simulink model "AIE_HLS"  (R2023a)
settings: Solver=FixedStepDiscrete  StartTime=0.0  StopTime=100*2e-9  RelTol=1e-3
undefined symbols (not defined in the file): i, L, nsvg1369, xcvc1502
libraries: dspsrcs4 x3, aieBasic x3, hlsBasic x2, vmcUtilities x1
settings Model: Creator=shirazi  LastModifiedBy=robg
settings SolverCC: AlgebraicLoopSolver=TrustRegion
settings DebuggingCC: UnconnectedInputMsg=warning  UnconnectedOutputMsg=warning  UnconnectedLineMsg=warning
settings ModelReferenceCC: EnableRefExpFcnMdlSchedulingChecks=on
settings SFSimCC: CustomCodeUndefinedFunction=UseInterfaceOnly
settings RTWCC: DLArmComputeVersion=19.05

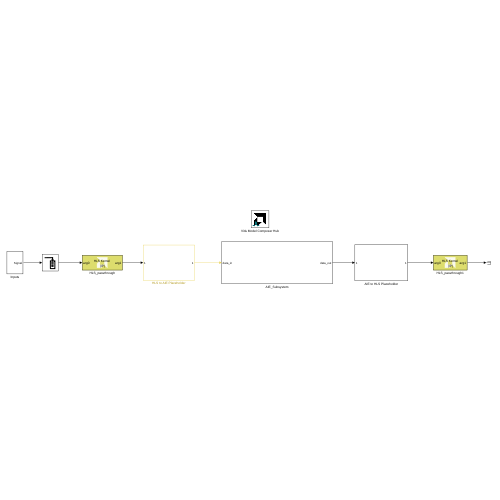
[thumbnail: Simulink's stored preview of the top-level diagram]
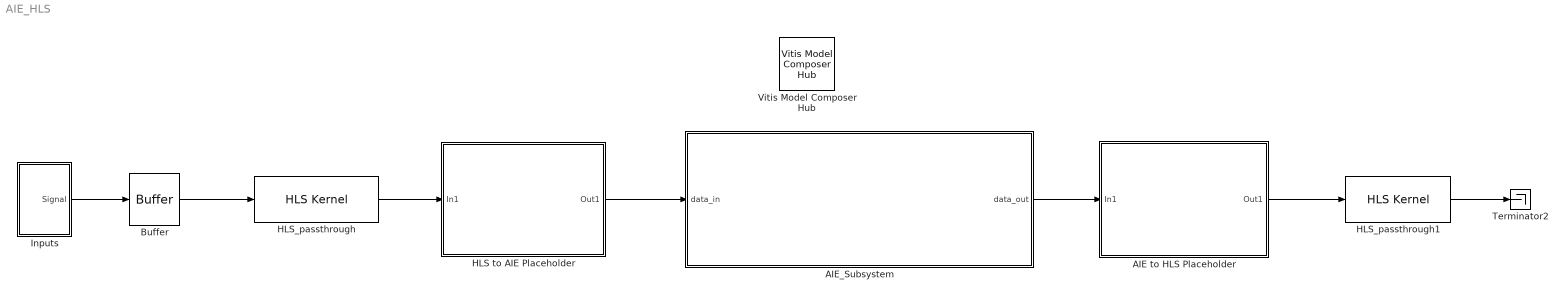
== system AIE_HLS ==
  AIE to HLS Placeholder : Subsystem
  AIE_Subsystem : Subsystem
  Buffer : Buffer  N=8  OutputFrames=off
  HLS to AIE Placeholder : Subsystem
  HLS_passthrough : hlsBasic/HLS Kernel  PortNames={'return'; 'arg0'; 'arg1'}  PortSerializedTypes={'{Bv}'; '{R{Thls::stream{2{t{Bu64t}}{t{}0}}}}'; '{R{Thls::stream{2{t{Bu64t}}{t{}0}}}}'}  FunctionTemplateSpecKind=none  FunctionTemplateParamNames={}  FunctionTemplateParamKinds={}  FunctionTemplateParamTypes={}  FunctionTemplateParamValues={}  PortSynchronicities={'auto'; 'auto'}  PortSignalSizes={0.000000000000000000e+00; 8.000000000000000000e+00}  PortParameterValues={}  FunctionTemplateParams={}  FunctionTemplateParamsEnables={}  FunctionTemplateParamsVisible=off  FunctionDeclTypeOptions=C[1 1]@t7@<empty>  PortAttributesTable={ 'Input', 'arg0', 'hls::stream< uint64_t, 0 > &', '', ''; 'Output', 'arg1', 'hls::stream< uint64_t, 0 > &', '', '8' }  PortAttributesEnablement={'off', 'off', 'off', 'off', 'off';'off', 'off', 'off', 'off', 'on'}  PortParametersTable={}  SampleTime=-1  PortDirectionTable={ 'arg0', 'hls::stream< uint64_t, 0 > &', 'Input', 'Port'; 'arg1', 'hls::stream< uint64_t, 0 > &', 'Output', 'Port' }  PortDirectionTabVisible=on  ArgDirections={1.000000000000000000e+00; 2.000000000000000000e+00}  ArgInterfaceTypes={1.000000000000000000e+00; 1.000000000000000000e+00}  FunctionIndex=1  FormalArgDecls={'hls::stream< uint64_t, 0 > & arg0', 'hls::stream< uint64_t, 0 > & arg1'}  SimLibPath=''  FunctionTabVisible=on  FunctionDescription=void HLS_passthrough(hls::stream< uint64_t, 0 > & arg0, hls::stream< uint64_t, 0 > & arg1)  blockJsonConstraints=[]  deprecateConstraints=0  KernelHeaderFile=HLS_passthrough.h  KernelFunction=HLS_passthrough  KernelFunctionSelect=<empty>  KernelSourceFile=HLS_passthrough.cpp  KernelSearchPaths={}  PreProcOptions={}
  HLS_passthrough1 : hlsBasic/HLS Kernel  PortNames={'return'; 'arg0'; 'arg1'}  PortSerializedTypes={'{Bv}'; '{R{Thls::stream{2{t{Bu64t}}{t{}0}}}}'; '{R{Thls::stream{2{t{Bu64t}}{t{}0}}}}'}  FunctionTemplateSpecKind=none  FunctionTemplateParamNames={}  FunctionTemplateParamKinds={}  FunctionTemplateParamTypes={}  FunctionTemplateParamValues={}  PortSynchronicities={'auto'; 'auto'}  PortSignalSizes={0.000000000000000000e+00; 8.000000000000000000e+00}  PortParameterValues={}  FunctionTemplateParams={}  FunctionTemplateParamsEnables={}  FunctionTemplateParamsVisible=off  FunctionDeclTypeOptions=C[1 1]@t7@<empty>  PortAttributesTable={ 'Input', 'arg0', 'hls::stream< uint64_t, 0 > &', '', ''; 'Output', 'arg1', 'hls::stream< uint64_t, 0 > &', '', '8' }  PortAttributesEnablement={'off', 'off', 'off', 'off', 'off';'off', 'off', 'off', 'off', 'on'}  PortParametersTable={}  SampleTime=-1  PortDirectionTable={ 'arg0', 'hls::stream< uint64_t, 0 > &', 'Input', 'Port'; 'arg1', 'hls::stream< uint64_t, 0 > &', 'Output', 'Port' }  PortDirectionTabVisible=on  ArgDirections={1.000000000000000000e+00; 2.000000000000000000e+00}  ArgInterfaceTypes={1.000000000000000000e+00; 1.000000000000000000e+00}  FunctionIndex=1  FormalArgDecls={'hls::stream< uint64_t, 0 > & arg0', 'hls::stream< uint64_t, 0 > & arg1'}  SimLibPath=''  FunctionTabVisible=on  FunctionDescription=void HLS_passthrough(hls::stream< uint64_t, 0 > & arg0, hls::stream< uint64_t, 0 > & arg1)  blockJsonConstraints=[]  deprecateConstraints=0  KernelHeaderFile=HLS_passthrough.h  KernelFunction=HLS_passthrough  KernelFunctionSelect=<empty>  KernelSourceFile=HLS_passthrough.cpp  KernelSearchPaths={}  PreProcOptions={}
  Inputs : Subsystem
  Terminator2 : Terminator
  Vitis Model Composer Hub : vmcUtilities/Vitis Model Composer Hub  Tag=genX  CodeGeneration=off  StartColumn=1  NumberOfColumns=1  TargetDirectory=./code  exportDesign=off  analyzeDesign=off  validateDesignOnHw=off  ExportType=AI Engines  IpVendor=xilinx.com  IpLibrary=hls  IpVersion=1.0  IpHWLanguage=Verilog  AieCompilerOptions={}  AieSimulatorOptions={}  CreateTestbench=off  TestbenchStackSize=10  RunRtlSim=off  RunCSim=off  RunAieSim=off  AieSimTimeout=50000  RunAieSimProfiling=off  LaunchVitisAnalyzer=off  PlotOutput=off  RunX86Sim=off  X86SimTimeout=10  GenHwImage=off  GenLibadfXo=off  GenHwValidationCode=off  PlatformType=Not Specified  HwSystemType=Baremetal  HwValidationTarget=hw  ProjDevice=xcvc1502-nsvg1369-1LHP-i-L  ProjDevicePart=xcvc1502-nsvg1369-1LHP-i-L  AIEType=AIE  SamplePeriod=-1  ClockFrequency=200  DataPathParallelism=1  xilinxfamily=versalaicore  part=xcvc1502  speed=-1LHP-i-L  package=nsvg1369  directory=./code  testbench=off  incr_netlist=off  synthesis_tool=Vivado  clock_wrapper=Clock Enables  dbl_ovrd=According to Block Masks  dcm_input_clock_period=10  sysclk_period=10  simulink_period=1  eval_field=0  LogFileName=''  NThreads=4
  wires:
  HLS to AIE Placeholder/1(Out1) -> AIE_Subsystem/1(data_in)
  AIE_Subsystem/1(data_out) -> AIE to HLS Placeholder/1(In1)
  Inputs/1(Signal) -> Buffer/1
  HLS_passthrough1/1 -> Terminator2/1
  AIE to HLS Placeholder/1(Out1) -> HLS_passthrough1/1
  HLS_passthrough/1 -> HLS to AIE Placeholder/1(In1)
  Buffer/1 -> HLS_passthrough/1

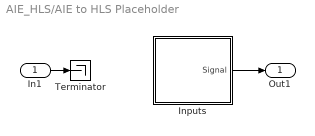
== system AIE_HLS/AIE to HLS Placeholder ==
  In1 : Inport
  Inputs : Subsystem
  Terminator : Terminator
  Out1 : Outport
  wires:
  Inputs/1(Signal) -> Out1/1
  In1/1 -> Terminator/1

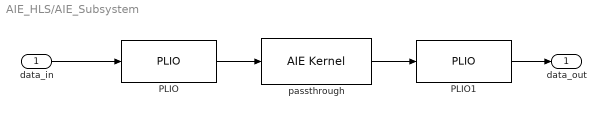
== system AIE_HLS/AIE_Subsystem ==
  data_in : Inport
  PLIO : aieBasic/PLIO  PlioWidth=64  PlioFreqSpec=on  PlioFreq=500  ColLocation=0  channel=0  blockJsonConstraints=[]  deprecateConstraints=0
  PLIO1 : aieBasic/PLIO  PlioWidth=64  PlioFreqSpec=on  PlioFreq=500  ColLocation=0  channel=0  blockJsonConstraints=[]  deprecateConstraints=0
  passthrough : aieBasic/AIE Kernel  KernelAllAttrs=|  PortNames={'in'; 'out'}  PortSerializedTypes={'{R{Tadf::input_buffer{1{t{Scint16}}}}}'; '{R{Tadf::output_buffer{1{t{Scint16}}}}}'}  PortWindowSizes={1.600000000000000000e+01, 1.600000000000000000e+01}  PortWindowMargins={0.000000000000000000e+00, 0.000000000000000000e+00}  PortSynchronicities={'sync', 'sync'}  PortSignalSizes={0.000000000000000000e+00; 0.000000000000000000e+00}  FunctionTemplateSpecKind=implicit  FunctionTemplateParamNames={'FRAME_LENGTH'}  FunctionTemplateParamKinds={'nontype'}  FunctionTemplateParamTypes={'int'}  FunctionTemplateParamValues={'16'}  FunctionIndex=1  FunctionTabVisible=on  FunctionTemplateParamsVisible=on  FunctionDeclTypeOptions=|  FunctionDecl=|  FunctionTemplateParams={ 'FRAME_LENGTH', 'int', '16' }  FunctionTemplateParamsEnables={'off', 'off', 'on'}  PortAttrs={ 'input', 'in', 'adf::input_buffer< cint16 > &', '16', '0', 'sync', ''; 'output', 'out', 'adf::output_buffer< cint16 > &', '16', '', 'sync', '' }  PortAttrsEnables={'off', 'off', 'off', 'on', 'off', 'off', 'off';'off', 'off', 'off', 'on', 'off', 'off', 'off'}  SampleTime=-1  KernelHeaderFile=passthrough.h  KernelFunction=passthrough  KernelSourceFile=passthrough.cc  KernelSearchPaths={}  PreProcOptions={}  blockJsonConstraints=[]
      KernelAllAttrs=|
      | s[12;12;9;9;19;14;21;23;21;23;24;21;15;17;12;24;26;26;26;27;28;9;21;23;23;23;24;25;14;19;19;29]@FunctionNameDeclFileNamePortNamesPortTypesPortSerializedTypesPortDirectionsPortWindowSizeEnablesPortWindowMarginEnablesPortBufferSizeEnablesPortBufferMarginEnablesPortSynchronicityEnablesPortSignalSizeEnablesPortBufferSizesPortBufferMarginsFunctionDeclFunctionTemplateSpecKindFunctionTemplateParamNamesFunctionTemplateParamKindsFunctionTemplateParamTypesFunctionTemplateParamValuesFunctionTemplateParamEnablesClassDeclClassTemplateSpecKindClassTemplateParamNamesClassTemplateParamKindsClassTemplateParamTypesClassTemplateParamValuesClassTemplateParamEnablesClassCtorDeclsClassCtorParamNamesClassCtorParamTypesClassCtorParamSerializedTypes[1 1]@C[32 1]@t11@passthrought19@../../passthrough.hC[2 1]@t2@int3@outC[2 1]@t29@adf::input_buffer< cint16 > &t30@adf::output_buffer< cint16 > &C[2 1]@t38@{R{Tadf::input_buffer{1{t{Scint16}}}}}t39@{R{Tadf::output_buffer{1{t{Scint16}}}}}C[2 1]@t5@inputt6@outputC[2 1]@l1@l1@C[2 1]@l1@l0@C[2 1]@l1@l1@C[2 1]@l0@l0@C[2 1]@l1@l1@C[2 1]@l0@l0@C[2 1]@nnC[2 1]@nnt117@template < int FRAME_LENGTH > 
      | void passthrough(adf::input_buffer< cint16 > & in, adf::output_buffer< cint16 > & out)t8@implicitC[1 1]@t12@FRAME_LENGTHC[1 1]@t7@nontypeC[1 1]@t3@intC[1 1]@nC[1 1]@l1@nne[0 1]@e[0 1]@e[0 1]@e[0 1]@e[0 1]@e[0 1]@e[0 1]@e[0 1]@e[0 1]@
      FunctionDeclTypeOptions=|
      | C[1 1]@t119@template < int FRAME_LENGTH > 
      | void passthrough(adf::input_buffer< cint16 > && in, adf::output_buffer< cint16 > && out)
      FunctionDecl=|
      | template < int FRAME_LENGTH > 
      | void passthrough(adf::input_buffer< cint16 > && in, adf::output_buffer< cint16 > && out)
  data_out : Outport
  wires:
  data_in/1 -> PLIO/1
  passthrough/1 -> PLIO1/1
  PLIO/1 -> passthrough/1
  PLIO1/1 -> data_out/1

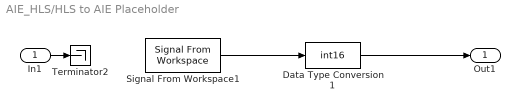
== system AIE_HLS/HLS to AIE Placeholder ==
  In1 : Inport
  Data Type Conversion1 : DataTypeConversion  OutDataTypeStr=int16  SaturateOnIntegerOverflow=off  RndMeth=Floor
  Signal From Workspace1 : dspsrcs4/Signal From Workspace  X=complex(1:100,1:100)  Ts=(2e-9)/2  nsamps=16  OutputAfterFinalValue=Cyclic repetition  ignoreOrWarnInputAndFrameLengths=off  OutputFrames=off
  Terminator2 : Terminator
  Out1 : Outport
  wires:
  Signal From Workspace1/1 -> Data Type Conversion1/1
  In1/1 -> Terminator2/1
  Data Type Conversion1/1 -> Out1/1

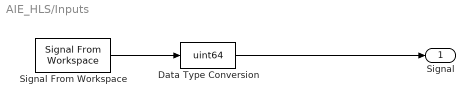
== system AIE_HLS/Inputs ==
  Data Type Conversion : DataTypeConversion  OutDataTypeStr=uint64  SaturateOnIntegerOverflow=off  RndMeth=Floor
  Signal From Workspace : dspsrcs4/Signal From Workspace  X=1:100  Ts=2e-9  nsamps=1  OutputAfterFinalValue=Cyclic repetition  ignoreOrWarnInputAndFrameLengths=off  OutputFrames=off
  Signal : Outport
  wires:
  Data Type Conversion/1 -> Signal/1
  Signal From Workspace/1 -> Data Type Conversion/1

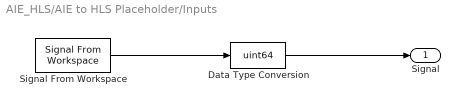
== system AIE_HLS/AIE to HLS Placeholder/Inputs ==
  Data Type Conversion : DataTypeConversion  OutDataTypeStr=uint64  SaturateOnIntegerOverflow=off  RndMeth=Floor
  Signal From Workspace : dspsrcs4/Signal From Workspace  X=1:100  Ts=(2e-9)  nsamps=8  OutputAfterFinalValue=Cyclic repetition  ignoreOrWarnInputAndFrameLengths=off  OutputFrames=off
  Signal : Outport
  wires:
  Signal From Workspace/1 -> Data Type Conversion/1
  Data Type Conversion/1 -> Signal/1
